simulink model "GFLIB_AtanYXShifted_BAM"  (Simulink 9.3)
settings: Solver=VariableStepAuto  StartTime=0.0  StopTime=10.0  RelTol=1e-3
settings Model: Creator=nxa18952  LastModifiedBy=nxa18952
settings DataIOCC: SaveFormat=Dataset  SignalLoggingSaveFormat=Dataset  ReturnWorkspaceOutputs=on
settings OptimizationCC: LifeSpan=auto
settings DebuggingCC: UnderspecifiedInitializationDetection=Simplified  MergeDetectMultiDrivingBlocksExec=error  FcnCallInpInsideContextMsg=error  SFUnexpectedBacktrackingDiag=error  SFNoUnconditionalDefaultTransitionDiag=error  SFExecutionAtInitializationDiag=warning  ArithmeticOperatorsInVariantConditions=error
settings HardwareCC: ProdBitPerPointer=64  ProdBitPerSizeT=64  ProdBitPerPtrDiffT=64  ProdLargestAtomicFloat=Float  ProdIntDivRoundTo=Zero  ProdEndianess=LittleEndian  ProdWordSize=64  ProdHWDeviceType=Intel->x86-64 (Windows64)
settings ModelReferenceCC: PropagateSignalLabelsOutOfModel=on
settings SFSimCC: SimUseLocalCustomCode=on
settings RTWCC: RTWUseLocalCustomCode=on
settings CodeAppCC: StateflowObjectComments=off
settings GRTTargetCC: TargetLangStandard=C99 (ISO)  CombineOutputUpdateFcns=on  GRTInterface=off
settings ConfigComp: CovMetricSettings=dwe  CovHtmlReporting=off  CovSaveCumulativeToWorkspaceVar=off  CovSaveSingleToWorkspaceVar=off  CovExternalEMLEnable=on

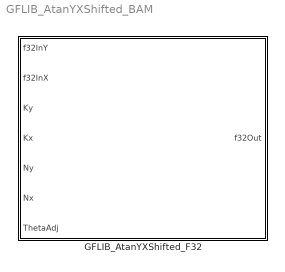
== system GFLIB_AtanYXShifted_BAM ==
  GFLIB_AtanYXShifted_F32 : Subsystem  TreatAsAtomicUnit=on  mask(GFLIB_AtanYXShifted_F32){}
      mask help: Shifted arctangent of two arguments Y/X in 32-bit fixed-point fractional implementation. Refer to the AMMCLIB User's Guide for further details.
      mask init:
      | if ~evalin('base','exist(''tS8'',''var'')')
      |   if (2 ~= exist('SWLIBS_Typedefs.mat','file'))
      |       error('File SWLIBS_Typedefs.mat is not on the Matlab path. Please add the AMMCLIB "bam" folder in the Matlab Search Path.');
      |   else
      |       evalin('base', 'load(''SWLIBS_Typedefs.mat'')');
      |   end
      | end
      settings: RTWSystemCode=Inline
      mask Display: pos = get_param(gcb, 'Position');width = pos(3) - pos(1); height = pos(4) - pos(2);tX=width/2;tY=height - 8;color('black');text(tX,tY, 'GFLIB_AtanYXShifted_F32', 'horizontalAlignment', 'center');

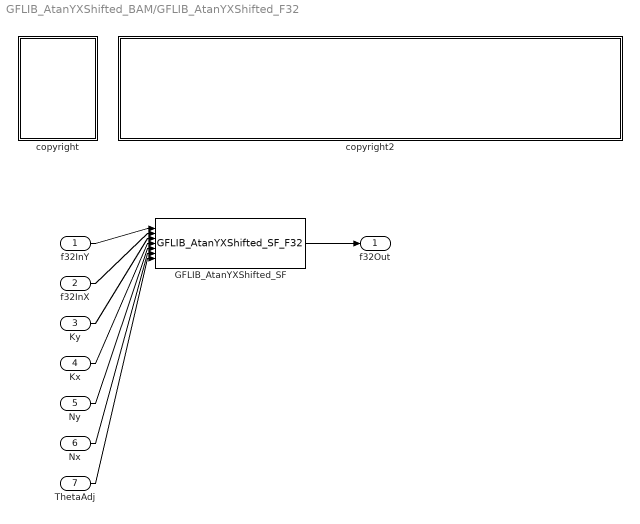
== system GFLIB_AtanYXShifted_BAM/GFLIB_AtanYXShifted_F32 ==
  f32InY : Inport  OutDataTypeStr=int32
  f32InX : Inport  Port=2  OutDataTypeStr=int32
  Ky : Inport  Port=3  OutDataTypeStr=int32
  Kx : Inport  Port=4  OutDataTypeStr=int32
  Ny : Inport  Port=5  OutDataTypeStr=int32
  Nx : Inport  Port=6  OutDataTypeStr=int32
  ThetaAdj : Inport  Port=7  OutDataTypeStr=int32
  GFLIB_AtanYXShifted_SF : S-Function  FunctionName=GFLIB_AtanYXShifted_SF_F32  SFunctionDeploymentMode=off  EnableBusSupport=off
  copyright : Subsystem
      mask Display: text(10,90,'FILE:');text(10,75,'DESRIPTION:');text(10,60,'COPYRIGHT:');text(10,45,'VERSION:');text(10,30,'DATE:')
  copyright2 : Subsystem
      mask Display: text(10,90,'GFLIB_AtanYXShifted_BAM_F32.mdl');text(10,75,'Shifted arctangent of two arguments Y/X.');text(10,60,'NXP 2020');text(10,45,'1.0');text(10,30,'18-Mar-2020');
  f32Out : Outport
  wires:
  f32InY/1 -> GFLIB_AtanYXShifted_SF/1
  f32InX/1 -> GFLIB_AtanYXShifted_SF/2
  Ky/1 -> GFLIB_AtanYXShifted_SF/3
  Kx/1 -> GFLIB_AtanYXShifted_SF/4
  Ny/1 -> GFLIB_AtanYXShifted_SF/5
  Nx/1 -> GFLIB_AtanYXShifted_SF/6
  ThetaAdj/1 -> GFLIB_AtanYXShifted_SF/7
  GFLIB_AtanYXShifted_SF/1 -> f32Out/1

== system GFLIB_AtanYXShifted_BAM/GFLIB_AtanYXShifted_F32/copyright ==

== system GFLIB_AtanYXShifted_BAM/GFLIB_AtanYXShifted_F32/copyright2 ==
